simulink model "modelo"  (Simulink 9.3)
settings: Solver=ode15s  StartTime=0.0  StopTime=inf  RelTol=1e-6  EnableMultiTasking=on
libraries: dspmathops x11, dsparch4 x10, dspvision x1, dspindex x1, dspobslib x1
settings Model: Creator=USUARIO  LastModifiedBy=Alfzzzzz
settings DataIOCC: LimitDataPoints=on  SignalLoggingName=sigsOut
settings OptimizationCC: ExpressionDepthLimit=2147483647  InitFltsAndDblsToZero=on
settings DebuggingCC: SaveWithParameterizedLinksMsg=none  SignalResolutionControl=TryResolveAllWithWarning  MultiTaskDSMMsg=warning  MultiTaskCondExecSysMsg=none  StateNameClashWarn=warning
settings HardwareCC: TargetUnknown=on
settings GRTTargetCC: TargetFcnLib=ansi_tfl_tmw.mat
settings ConfigComp: CovExternalEMLEnable=on

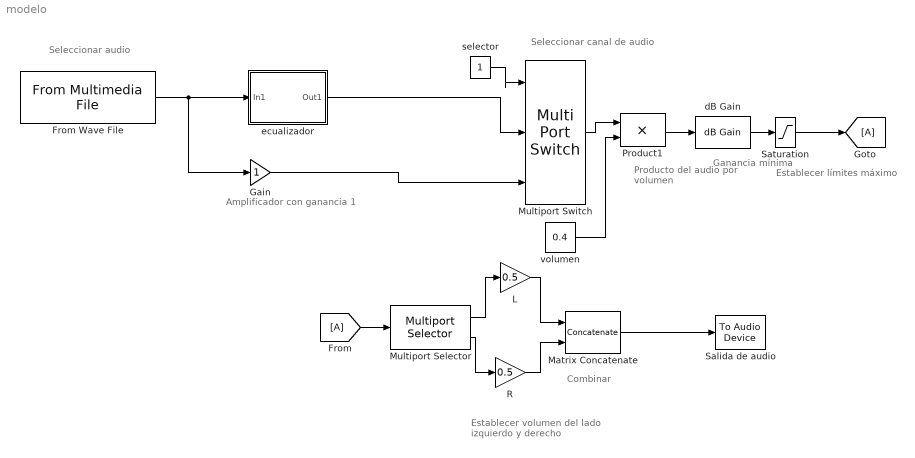
== system modelo ==
  note: Combinar
  note: Establecer volumen del lado izquierdo y derecho
  note: Establecer límites máximo
  note: Ganancia
      | mínima
  note: Producto del audio por volumen
  note: Amplificador con ganancia 1
  note: Seleccionar canal de audio
  note: Seleccionar audio
  From Wave File : dspvision/From Multimedia File  inputFilename=C:\Users\Alfzzzzz\Downloads\Ecualización\Mozart_stereo.wav  readRange=[1 Inf]  loop=on  numPlays=1  outputStreams=Audio only  videoDataType=single  audioDataType=double  inheritSampleTime=on  userDefinedSampleTime=1/30  noAudioOutput=off  isIntensityVideo=off  fourcc=RGB  colorVideoFormat=Separate color signals  outputEOF=off  dataOrg=Column-major  audioFrameSize=256  computeAudioFrameSize=off  outSamplingMode=Frame based
      settings: SourceProductName=DSP System Toolbox  SourceProductBaseCode=DS
  Gain : Gain
  L : Gain  Gain=0.5
  Matrix Concatenate : Concatenate  Mode=Multidimensional array  ConcatenateDimension=2
  Multiport Selector : dspindex/Multiport Selector  rowsOrCols=Columns  idxCellArray={1,2}  idxErrMode=Clip and Warn
  Multiport Switch : MultiPortSwitch  Inputs=2  SaturateOnIntegerOverflow=on
  Product1 : Product  SaturateOnIntegerOverflow=on  OutDataTypeStr=Inherit: Same as first input
  R : Gain  Gain=0.5
  Salida de audio : dspobslib/To Audio Device  deviceName=Default  inheritSampleRate=on  sampleRate=44100  deviceDatatype=Determine from input data type  autoBufferSize=on  bufferSize=4096  queueDuration=2  defaultOutputChannelMapping=on  outputChannelMapping=1:2  outputNumUnderrunSamples=off
      settings: SourceProductName=DSP System Toolbox  SourceProductBaseCode=DS
  Saturation : Saturate  UpperLimit=5  LowerLimit=-5  LinearizeAsGain=off  ZeroCross=off
  dB Gain : dspmathops/dB Gain  dB=5  intype=Amplitude
      settings: SourceProductName=DSP System Toolbox  SourceProductBaseCode=DS
  ecualizador : Subsystem
  selector : Constant
  volumen : Constant  Value=0.4
  wires:
  selector/1 -> Multiport Switch/1
  Multiport Switch/1 -> Product1/1
  Product1/1 -> dB Gain/1
  volumen/1 -> Product1/2
  dB Gain/1 -> Saturation/1
  Saturation/1 -> [A]
  From Wave File/1 -> Gain/1, ecualizador/1(In1)
  Multiport Selector/2 -> R/1
  Multiport Selector/1 -> L/1
  L/1 -> Matrix Concatenate/1
  R/1 -> Matrix Concatenate/2
  Matrix Concatenate/1 -> Salida de audio/1
  [A] -> Multiport Selector/1
  ecualizador/1(Out1) -> Multiport Switch/2
  Gain/1 -> Multiport Switch/3

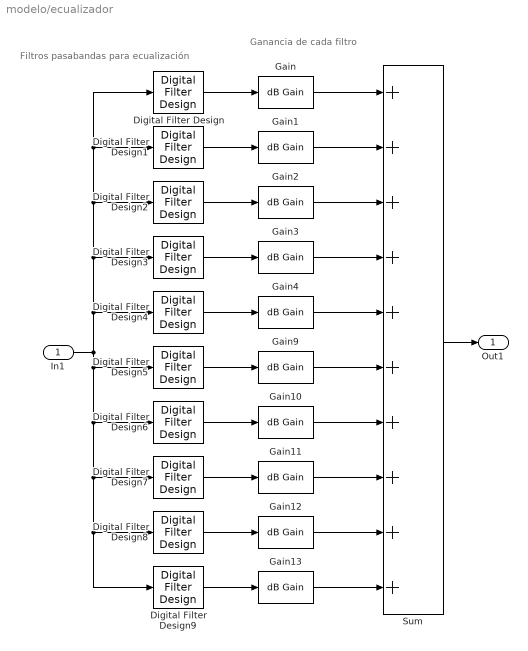
== system modelo/ecualizador ==
  note: Ganancia de cada filtro
  note: Filtros pasabandas para ecualización
  In1 : Inport
  Digital Filter Design{,1..9} (10 alike) : dsparch4/Digital Filter Design  mwdsp_browser_bugfix_var=off
  Gain : dspmathops/dB Gain  dB=4  intype=Amplitude
      settings: SourceProductName=DSP System Toolbox  SourceProductBaseCode=DS
  Gain1 : dspmathops/dB Gain  dB=3  intype=Amplitude
      settings: SourceProductName=DSP System Toolbox  SourceProductBaseCode=DS
  Gain10 : dspmathops/dB Gain  dB=4  intype=Amplitude
      settings: SourceProductName=DSP System Toolbox  SourceProductBaseCode=DS
  Gain{9,11..13} (4 alike) : dspmathops/dB Gain  dB=5  intype=Amplitude
      settings: SourceProductName=DSP System Toolbox  SourceProductBaseCode=DS
  Gain2 : dspmathops/dB Gain  dB=0  intype=Amplitude
      settings: SourceProductName=DSP System Toolbox  SourceProductBaseCode=DS
  Gain3 : dspmathops/dB Gain  dB=-2  intype=Amplitude
      settings: SourceProductName=DSP System Toolbox  SourceProductBaseCode=DS
  Gain4 : dspmathops/dB Gain  dB=-2  intype=Amplitude
      settings: SourceProductName=DSP System Toolbox  SourceProductBaseCode=DS
  Sum : Sum  Inputs=++++++++++  SaturateOnIntegerOverflow=on
  Out1 : Outport  VectorParamsAs1DForOutWhenUnconnected=on
  wires:
  In1/1 -> Digital Filter Design4/1, Digital Filter Design/1, Digital Filter Design1/1, Digital Filter Design2/1, Digital Filter Design3/1, Digital Filter Design5/1, Digital Filter Design6/1, Digital Filter Design7/1, Digital Filter Design9/1, Digital Filter Design8/1
  Sum/1 -> Out1/1
  Digital Filter Design/1 -> Gain/1
  Digital Filter Design1/1 -> Gain1/1
  Digital Filter Design2/1 -> Gain2/1
  Digital Filter Design3/1 -> Gain3/1
  Digital Filter Design4/1 -> Gain4/1
  Digital Filter Design5/1 -> Gain9/1
  Digital Filter Design6/1 -> Gain10/1
  Digital Filter Design7/1 -> Gain11/1
  Digital Filter Design8/1 -> Gain12/1
  Digital Filter Design9/1 -> Gain13/1
  Gain/1 -> Sum/1
  Gain1/1 -> Sum/2
  Gain2/1 -> Sum/3
  Gain3/1 -> Sum/4
  Gain4/1 -> Sum/5
  Gain9/1 -> Sum/6
  Gain10/1 -> Sum/7
  Gain11/1 -> Sum/8
  Gain12/1 -> Sum/9
  Gain13/1 -> Sum/10
